simulink model "LVS_model_upgrade"  (R2024b)
settings: Solver=FixedStepAuto  StartTime=0.0  StopTime=80  RelTol=1e-3
values from neighbouring files (symbols this model uses):
  AltitudeError = -65    [mc_light.m]    (also in scenario_settings.m)
  landmarks_initial = zeros(1, landmarks_number_lvs*10+1)    [mc_light.m]    (also in scenario_settings.m)
  Rand_x = -3000 + 6000*INIT_rand_values(6, run)    [mc_light.m]    (also in scenario_settings.m = -3000 + 6000*rand)
  Rand_y = -3000 + 6000*INIT_rand_values(7, run)    [mc_light.m]    (also in scenario_settings.m = -3000 + 6000*rand)
  ScalarError = sqrt(1-XAxisRotError^2-YAxisRotError^2-ZAxisRotError^2)    [mc_light.m]    (also in scenario_settings.m)
  Tl = 0.1    [main.m]    (also in mc_light.m)
  XAxisRotError = sin(PhiError/2)    [mc_light.m]    (also in scenario_settings.m)
  YAxisRotError = sin(ThtError/2)    [mc_light.m]    (also in scenario_settings.m)
  ZAxisRotError = sin(PsiError/2)    [mc_light.m]    (also in scenario_settings.m)
settings Model: Creator=alber  LastModifiedBy=Riccardo
settings DebuggingCC: UnconnectedInputMsg=warning  UnconnectedOutputMsg=warning  UnconnectedLineMsg=warning
settings ModelReferenceCC: EnableRefExpFcnMdlSchedulingChecks=on
settings RTWCC: GPUComputeCapability=3.5  DLArmComputeVersion=19.05

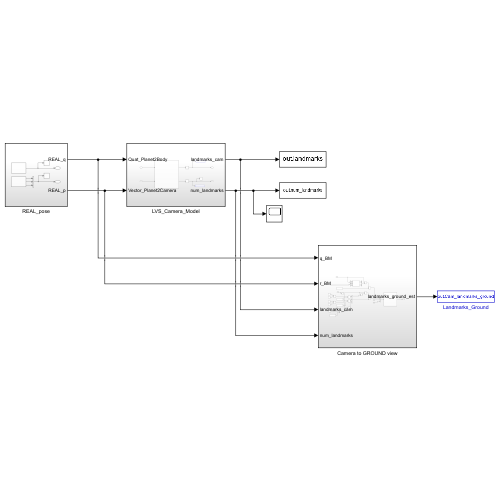
[thumbnail: Simulink's stored preview of the top-level diagram]
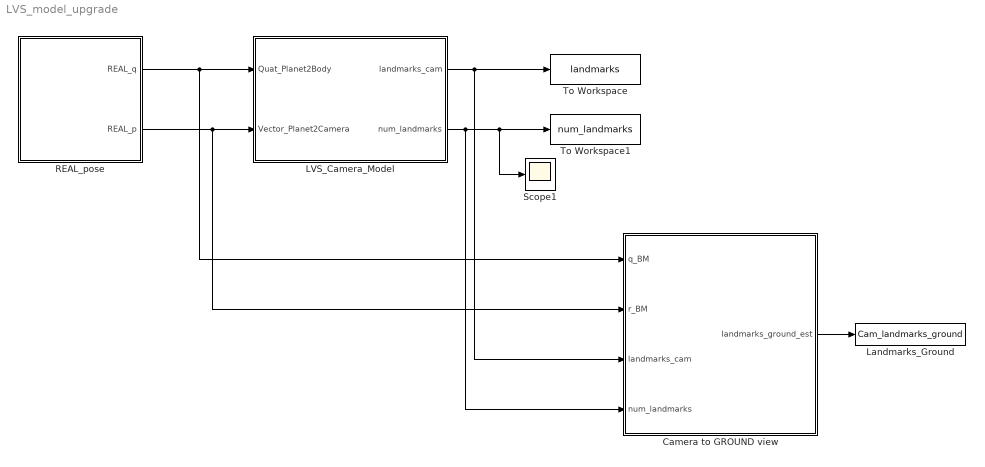
== system LVS_model_upgrade ==
  Camera to GROUND view : Subsystem
  LVS_Camera_Model : Subsystem
  Landmarks_Ground : ToWorkspace  VariableName=Cam_landmarks_ground  SampleTime=-1
  REAL_pose : Subsystem
  Scope1 : Scope
  To Workspace : ToWorkspace  VariableName=landmarks  SaveFormat=Timeseries  SampleTime=-1
  To Workspace1 : ToWorkspace  VariableName=num_landmarks  SampleTime=-1
  wires:
  REAL_pose/1(REAL_q) -> Camera to GROUND view/1(q_BM), LVS_Camera_Model/1(Quat_Planet2Body)
  LVS_Camera_Model/1(landmarks_cam) -> Camera to GROUND view/3(landmarks_cam), To Workspace/1
  LVS_Camera_Model/2(num_landmarks) -> Camera to GROUND view/4(num_landmarks), Scope1/1, To Workspace1/1
  REAL_pose/2(REAL_p) -> Camera to GROUND view/2(r_BM), LVS_Camera_Model/2(Vector_Planet2Camera)
  Camera to GROUND view/1(landmarks_ground_est) -> Landmarks_Ground/1

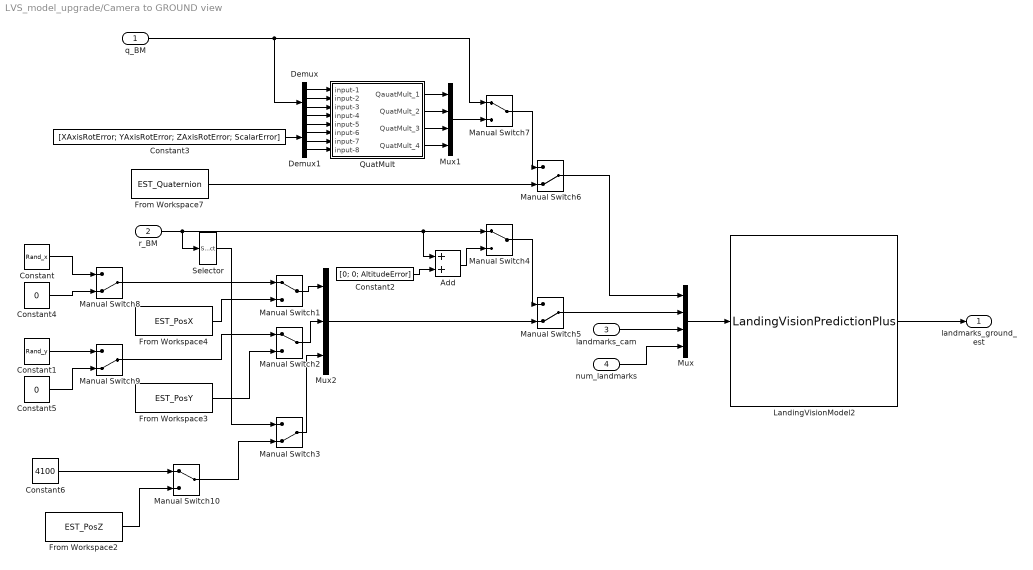
== system LVS_model_upgrade/Camera to GROUND view ==
  q_BM : Inport
  r_BM : Inport  Port=2
  landmarks_cam : Inport  Port=3
  num_landmarks : Inport  Port=4
  Add : Sum
  Constant : Constant  Value=Rand_x
  Constant1 : Constant  Value=Rand_y
  Constant2 : Constant  Value=[0; 0; AltitudeError]
  Constant3 : Constant  Value=[XAxisRotError; YAxisRotError; ZAxisRotError; ScalarError]
  Constant4 : Constant  Value=0
  Constant5 : Constant  Value=0
  Constant6 : Constant  Value=4100
  Demux : Demux
  Demux1 : Demux
  From Workspace2 : FromWorkspace  VariableName=EST_PosZ
  From Workspace3 : FromWorkspace  VariableName=EST_PosY
  From Workspace4 : FromWorkspace  VariableName=EST_PosX
  From Workspace7 : FromWorkspace  VariableName=EST_Quaternion
  LandingVisionModel2 : S-Function  FunctionName=LandingVisionPredictionPlus  Parameters=-1, r_CB, q_CB, w, h, actualf, n_points  SFunctionDeploymentMode=off  EnableBusSupport=off
  Manual Switch{1..2,4,7,10} (5 alike) : ManualSwitch
  Manual Switch{3,5..6,8..9} (5 alike) : ManualSwitch  CurrentSetting=0
  Mux : Mux
  Mux1 : Mux
  Mux2 : Mux  Inputs=3
  QuatMult : Subsystem
  Selector : Selector  InputPortWidth=3  IndexOptions=Index vector (dialog)  Indices=[3]  OutputSizes=1
  landmarks_ground_est : Outport
  wires:
  landmarks_cam/1 -> Mux/3
  Mux/1 -> LandingVisionModel2/1
  LandingVisionModel2/1 -> landmarks_ground_est/1
  num_landmarks/1 -> Mux/4
  q_BM/1 -> Demux/1, Manual Switch7/1
  Manual Switch5/1 -> Mux/2
  From Workspace4/1 -> Manual Switch1/2
  From Workspace2/1 -> Manual Switch10/2
  From Workspace3/1 -> Manual Switch2/2
  Mux2/1 -> Manual Switch5/2
  r_BM/1 -> Manual Switch4/1, Add/1, Selector/1
  From Workspace7/1 -> Manual Switch6/2
  Manual Switch6/1 -> Mux/1
  Manual Switch2/1 -> Mux2/2
  Manual Switch1/1 -> Mux2/1
  Constant1/1 -> Manual Switch9/1
  Constant/1 -> Manual Switch8/1
  Manual Switch3/1 -> Mux2/3
  Selector/1 -> Manual Switch3/1
  Add/1 -> Manual Switch4/2
  Constant2/1 -> Add/2
  Manual Switch4/1 -> Manual Switch5/1
  Manual Switch7/1 -> Manual Switch6/1
  Mux1/1 -> Manual Switch7/2
  Constant3/1 -> Demux1/1
  QuatMult/1(QauatMult_1) -> Mux1/1
  QuatMult/2(QuatMult_2) -> Mux1/2
  QuatMult/3(QuatMult_3) -> Mux1/3
  QuatMult/4(QuatMult_4) -> Mux1/4
  Demux/1 -> QuatMult/1(input-1)
  Demux/2 -> QuatMult/2(input-2)
  Demux/3 -> QuatMult/3(input-3)
  Demux/4 -> QuatMult/4(input-4)
  Demux1/1 -> QuatMult/5(input-5)
  Demux1/2 -> QuatMult/6(input-6)
  Demux1/3 -> QuatMult/7(input-7)
  Demux1/4 -> QuatMult/8(input-8)
  Manual Switch9/1 -> Manual Switch2/1
  Manual Switch8/1 -> Manual Switch1/1
  Constant4/1 -> Manual Switch8/2
  Constant5/1 -> Manual Switch9/2
  Constant6/1 -> Manual Switch10/1
  Manual Switch10/1 -> Manual Switch3/2

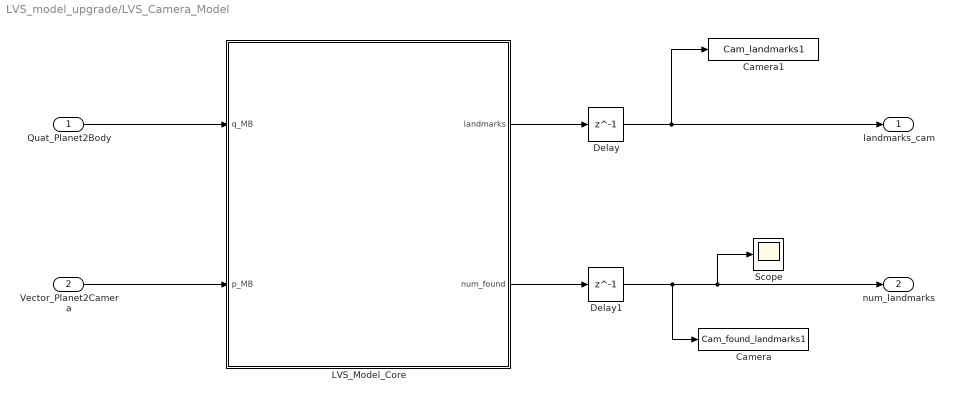
== system LVS_model_upgrade/LVS_Camera_Model ==
  Quat_Planet2Body : Inport
  Vector_Planet2Camera : Inport  Port=2
  Camera : ToWorkspace  VariableName=Cam_found_landmarks1  SampleTime=-1
  Camera1 : ToWorkspace  VariableName=Cam_landmarks1  SampleTime=-1
  Delay : Delay  DelayLength=1  InitialCondition=landmarks_initial  SampleTime=Tl
  Delay1 : Delay  DelayLength=1  InitialCondition=0  SampleTime=Tl
  LVS_Model_Core : Subsystem
  Scope : Scope
  landmarks_cam : Outport
  num_landmarks : Outport  Port=2
  wires:
  Delay1/1 -> Camera/1, num_landmarks/1, Scope/1
  LVS_Model_Core/1(landmarks) -> Delay/1
  Vector_Planet2Camera/1 -> LVS_Model_Core/2(p_MB)
  Delay/1 -> landmarks_cam/1, Camera1/1
  LVS_Model_Core/2(num_found) -> Delay1/1
  Quat_Planet2Body/1 -> LVS_Model_Core/1(q_MB)

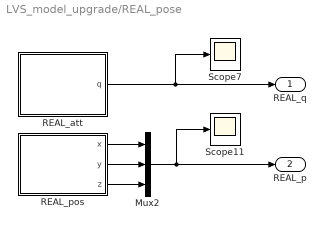
== system LVS_model_upgrade/REAL_pose ==
  Mux2 : Mux  Inputs=3
  REAL_att : Subsystem
  REAL_pos : Subsystem
  Scope11 : Scope
  Scope7 : Scope
  REAL_q : Outport
  REAL_p : Outport  Port=2
  wires:
  REAL_att/1(q) -> REAL_q/1, Scope7/1
  Mux2/1 -> REAL_p/1, Scope11/1
  REAL_pos/3(z) -> Mux2/3
  REAL_pos/1(x) -> Mux2/1
  REAL_pos/2(y) -> Mux2/2

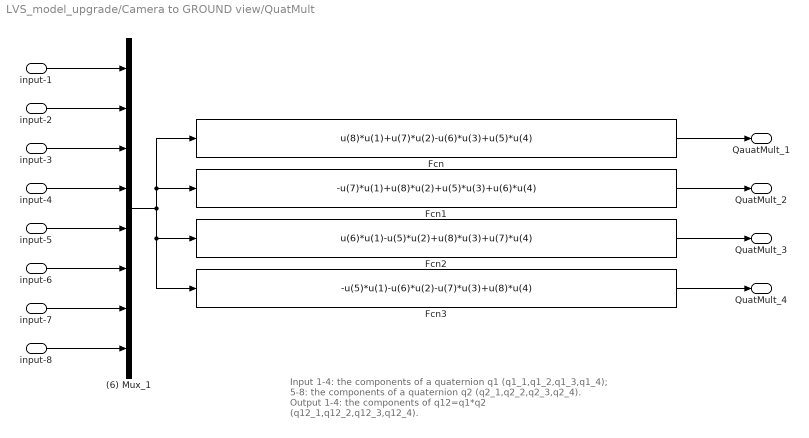
== system LVS_model_upgrade/Camera to GROUND view/QuatMult ==
  note: Input
      | 1-4: the components of a quaternion q1 (q1_1,q1_2,q1_3,q1_4);
      | 5-8: the components of a quaternion q2 (q2_1,q2_2,q2_3,q2_4).
      |
      | Output
      | 1-4: the components of q12=q1*q2 (q12_1,q12_2,q12_3,q12_4).
  input-1 : Inport
  input-2 : Inport  Port=2
  input-3 : Inport  Port=3
  input-4 : Inport  Port=4
  input-5 : Inport  Port=5
  input-6 : Inport  Port=6
  input-7 : Inport  Port=7
  input-8 : Inport  Port=8
  " (6) Mux_1" : Mux  Inputs=8
  Fcn : Fcn  Expr=u(8)*u(1)+u(7)*u(2)-u(6)*u(3)+u(5)*u(4)
  Fcn1 : Fcn  Expr=-u(7)*u(1)+u(8)*u(2)+u(5)*u(3)+u(6)*u(4)
  Fcn2 : Fcn  Expr=u(6)*u(1)-u(5)*u(2)+u(8)*u(3)+u(7)*u(4)
  Fcn3 : Fcn  Expr=-u(5)*u(1)-u(6)*u(2)-u(7)*u(3)+u(8)*u(4)
  QauatMult_1 : Outport
  QuatMult_2 : Outport  Port=2
  QuatMult_3 : Outport  Port=3
  QuatMult_4 : Outport  Port=4
  wires:
  " (6) Mux_1"/1 -> Fcn/1, Fcn1/1, Fcn3/1, Fcn2/1
  input-1/1 -> " (6) Mux_1"/1
  input-2/1 -> " (6) Mux_1"/2
  input-3/1 -> " (6) Mux_1"/3
  input-4/1 -> " (6) Mux_1"/4
  input-5/1 -> " (6) Mux_1"/5
  input-6/1 -> " (6) Mux_1"/6
  input-7/1 -> " (6) Mux_1"/7
  input-8/1 -> " (6) Mux_1"/8
  Fcn3/1 -> QuatMult_4/1
  Fcn2/1 -> QuatMult_3/1
  Fcn1/1 -> QuatMult_2/1
  Fcn/1 -> QauatMult_1/1

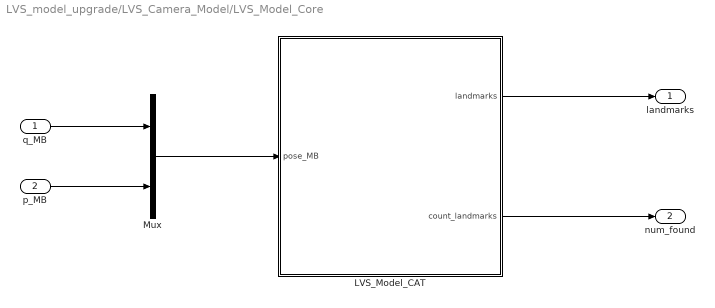
== system LVS_model_upgrade/LVS_Camera_Model/LVS_Model_Core ==
  q_MB : Inport
  p_MB : Inport  Port=2
  LVS_Model_CAT : Subsystem
  Mux : Mux  Inputs=2
  landmarks : Outport
  num_found : Outport  Port=2
  wires:
  LVS_Model_CAT/2(count_landmarks) -> num_found/1
  LVS_Model_CAT/1(landmarks) -> landmarks/1
  Mux/1 -> LVS_Model_CAT/1(pose_MB)
  q_MB/1 -> Mux/1
  p_MB/1 -> Mux/2

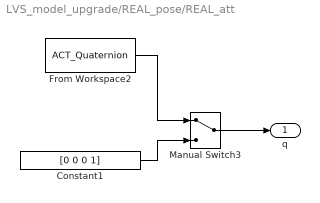
== system LVS_model_upgrade/REAL_pose/REAL_att ==
  Constant1 : Constant  Value=[0 0 0 1]
  From Workspace2 : FromWorkspace  VariableName=ACT_Quaternion
  Manual Switch3 : ManualSwitch
  q : Outport
  wires:
  Constant1/1 -> Manual Switch3/2
  Manual Switch3/1 -> q/1
  From Workspace2/1 -> Manual Switch3/1

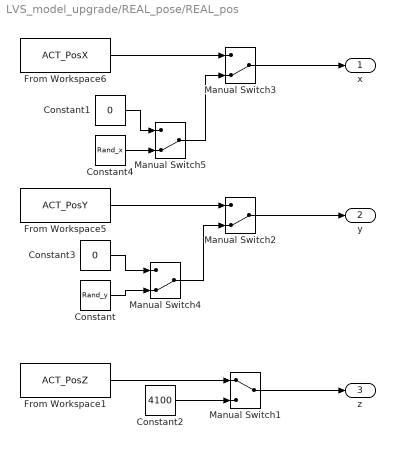
== system LVS_model_upgrade/REAL_pose/REAL_pos ==
  Constant : Constant  Value=Rand_y
  Constant1 : Constant  Value=0
  Constant2 : Constant  Value=4100
  Constant3 : Constant  Value=0
  Constant4 : Constant  Value=Rand_x
  From Workspace1 : FromWorkspace  VariableName=ACT_PosZ
  From Workspace5 : FromWorkspace  VariableName=ACT_PosY
  From Workspace6 : FromWorkspace  VariableName=ACT_PosX
  Manual Switch1 : ManualSwitch
  Manual Switch{2..5} (4 alike) : ManualSwitch  CurrentSetting=0
  x : Outport
  y : Outport  Port=2
  z : Outport  Port=3
  wires:
  Manual Switch1/1 -> z/1
  Constant2/1 -> Manual Switch1/2
  From Workspace6/1 -> Manual Switch3/1
  From Workspace1/1 -> Manual Switch1/1
  From Workspace5/1 -> Manual Switch2/1
  Manual Switch3/1 -> x/1
  Manual Switch2/1 -> y/1
  Constant1/1 -> Manual Switch5/1
  Constant3/1 -> Manual Switch4/1
  Constant/1 -> Manual Switch4/2
  Manual Switch4/1 -> Manual Switch2/2
  Constant4/1 -> Manual Switch5/2
  Manual Switch5/1 -> Manual Switch3/2

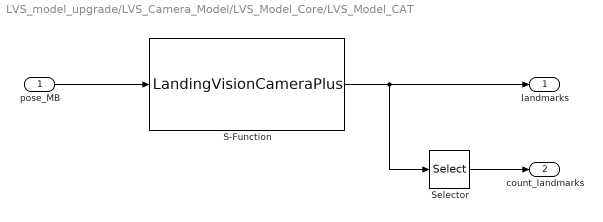
== system LVS_model_upgrade/LVS_Camera_Model/LVS_Model_Core/LVS_Model_CAT ==
  pose_MB : Inport
  S-Function : S-Function  FunctionName=LandingVisionCameraPlus  Parameters=Tl, Cat, r_CB, q_CB, w, h, actualf, n_points  SFunctionDeploymentMode=off  EnableBusSupport=off
  Selector : Selector  InputPortWidth=1001  IndexOptions=Index vector (dialog)  Indices=[201]  OutputSizes=1
  landmarks : Outport
  count_landmarks : Outport  Port=2
  wires:
  Selector/1 -> count_landmarks/1
  S-Function/1 -> Selector/1, landmarks/1
  pose_MB/1 -> S-Function/1
